simulink model "PVAndBatteryIntegratedPlantForBlackStart"  (R2025b)
settings: Solver=FixedStepAuto  StartTime=0.0  StopTime=tsim  FixedStep=1e-6  RelTol=1e-9  AbsTol=1e-7
InitFcn:
  | %% Black Start Sequence
  | t0 = 0; % Battery IBR initial time
  | t1 = 0.15; % PV IBR initial time
  | t2 = 0.5; % Two IBR sync time
  | t3 = 0.8; % Additional motor load connect
  | t4 = 1.1; % Grid reconnection
  | tsim = 1.5; % Total simulation time
  | 
  | %% initialize
  | Vdc = 400;
  | Vnom = 100;
  | Prated = 10000;
  | Qrated = 0;
  | Srated = sqrt(Prated^2+Qrated^2);
  | wnom = 2*pi*60;
  | fnom = 60;
  | Vminpu = 0.95;
  | 
  | kv = Vnom;
  | ki = 3*Vnom/Srated;
  | 
  | dwmax = 0.5*2*pi;
  | trisemax = 0.1;
  | 
  | C = 1/sqrt(2)/Vminpu^2/dwmax;
  | L = 1/C/wnom^2;
  | tau = C/kv/ki;
  | epsilon = sqrt(L/C);
  | ksy = 3/2/trisemax;
  | 
  | V_voc_1 = 0;
  | V_voc_2 = 0;
  | 
  | % filter
  | Rf = 0.05;
  | Lf = 500e-6;
  | % pwm
  | fsw = 10e3;
  | % simulation
  | Ts = 1e-6;
  | 
  | % load
  | Rl = 3*Vnom^2/Prated;
  | Rl1 = Rl;
  | Rl2 = 2*Rl;
  | Rl3 = 20*Rl;
  | % grid
  | Rg = 0.05;
  | Lg = 50e-6;
  | 
  | % DCDC converter
  | Kp_V = 1;
  | Ki_V = 0.02;
  | Imax = 110;
  | Kp_I = 0.0001;
  | Ki_I = 1;
  | Vcmax = 1;
undefined symbols (not defined in the file): alpha, C_voc, Diode_class, Half_BridgeConverter_class, L_voc, Ll, Mosfet_class, PWMGenerator_DC_DC__class, R_voc, Three_PhaseBreaker_class, Three_PhaseSource_class, Three_PhaseTransformer_2_class, Three_PhaseV_IMeasuremen_class
libraries: nesl_utility x69, ee_lib x49, fl_lib x36, mcbeeMathTransformLib x9, simulink x6, spsParallelRLCBranchLib x3, eePwmGeneratorTwoLevel x2, spsControlledCurrentSourceLib x2, elec_conv_HighZElecRef x2, slpidlib x2, spsSecondOrderFilterLib x1, spsCurrentMeasurementLib x1
(part 1 of 4)
settings Model: SimulationMode=accelerator  Creator=marco  LastModifiedBy=marco
settings DebuggingCC: AlgebraicLoopMsg=none  SaveWithParameterizedLinksMsg=none
settings RTWCC: GPUComputeCapability=3.5

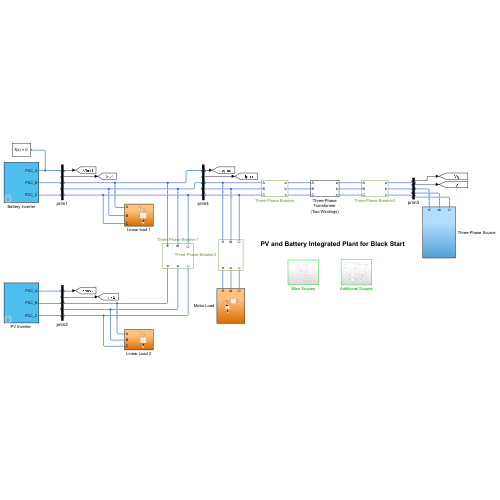
[thumbnail: Simulink's stored preview of the top-level diagram]
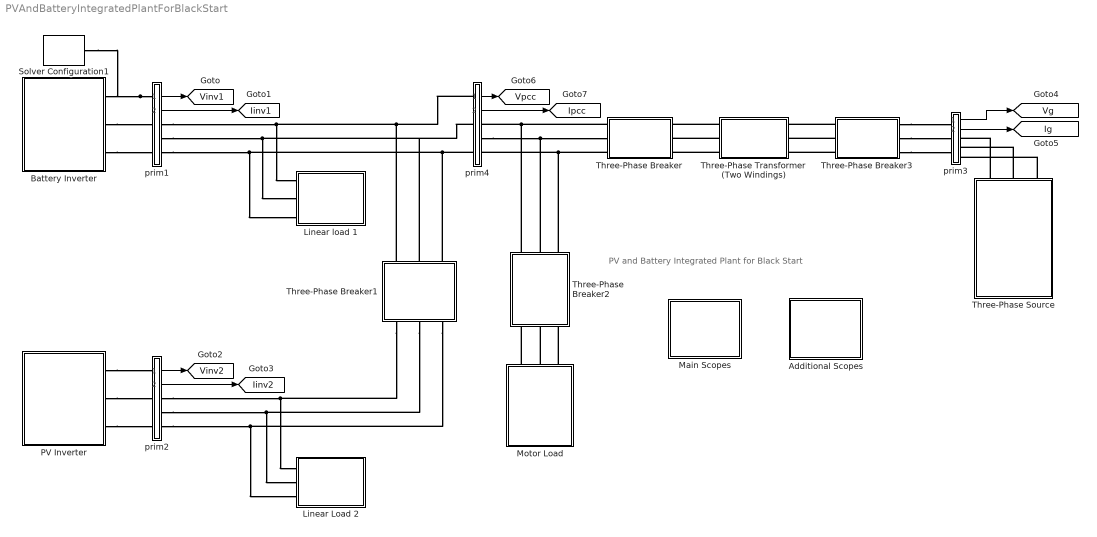
== system PVAndBatteryIntegratedPlantForBlackStart ==
  note: PV and Battery Integrated Plant for Black Start
  Additional Scopes : Subsystem
  Battery Inverter : Subsystem
      mask DialogControl DescTextVar Prompt: This is an IBR with battery source.
  Linear Load 2 : Subsystem
  Linear load 1 : Subsystem
  Main Scopes : Subsystem
  Motor Load : Subsystem
  "PV Inverter " : Subsystem
      mask DialogControl DescTextVar Prompt: This is an IBR with PV source.
  Solver Configuration1 : nesl_utility/Solver Configuration  PhysicalDomain=network_engine_domain  SubClassName=solver  LeftPortType=input  RightPortType=generic  Tones=[]  Harmonics=[]  SimulateNoise=off  Profile=off  UseLocalSampling=off  EnableSwitchedLinearOptims=on  FrequencyDomain=off  UseCCode=off  RelTol=0.001  AbsTol=0.001  MinStep=1e-09  ToWorkspace=off  RevertToSquareIcSolve=off  NumHomotopyIterations=100  PhasorMode=off  PhasorModeNumHarmonics=1  ConsistencySolver=NEWTON_XTOL_AFTER_FTOL  IndexReductionMethod=DerivativeReplacement  DoDC=off  ResidualTolerance=1e-09  ConsistencyTolSource=GLOBAL  ConsistencyAbsTol=0.001  ConsistencyRelTol=0.001  ConsistencyTolFactor=0.001  UseLocalSolver=off  LocalSolverChoice=NE_BACKWARD_EULER_ADVANCER  ResolveIndetEquations=on  FunctionEvalNumThread=1  LocalSolverSampleTime=1e-6  DoFixedCost=on  MaxNonlinIter=3  MaxModeIter=2  ComputeImpulses=off  ImpulseIterations=2  LinearAlgebra=auto  LinearAlgebraNumThread=0  EquationFormulation=NE_TIME_EF  DelaysMemoryBudget=1024  AutomaticFiltering=on  FilteringTimeConstant=0.001  PartitionStorageMethod=AS_NEEDED  PartitionMemoryBudget=1024  PartitionMethod=ROBUST  MultibodyUseLocalSolver=off  MultibodyLocalSolverChoice=ODE1  MultibodyLocalSolverSampleTime=0.001
  Three-Phase Transformer (Two Windings) : Subsystem
      settings: OpenFcn=elec.conv.unmask(gcb);
  Three-Phase Breaker : Subsystem
      settings: OpenFcn=elec.conv.unmask(gcb);
  Three-Phase Breaker1 : Subsystem
      settings: OpenFcn=elec.conv.unmask(gcb);
  Three-Phase Breaker2 : Subsystem
      settings: OpenFcn=elec.conv.unmask(gcb);
  Three-Phase Breaker3 : Subsystem
      settings: OpenFcn=elec.conv.unmask(gcb);
  Three-Phase Source : Subsystem
  prim1 : Subsystem
      settings: OpenFcn=elec.conv.unmask(gcb);
  prim2 : Subsystem
      settings: OpenFcn=elec.conv.unmask(gcb);
  prim3 : Subsystem
      settings: OpenFcn=elec.conv.unmask(gcb);
  prim4 : Subsystem
      settings: OpenFcn=elec.conv.unmask(gcb);
  tag scope: Ig=global, Iinv1=global, Iinv2=global, Ipcc=global, Vg=global, Vinv1=global, Vinv2=global, Vpcc=global
  wires:
  prim1/1(Vabc) -> [Vinv1]
  prim1/2(Iabc) -> [Iinv1]
  prim3/1(Vabc) -> [Vg]
  prim3/2(Iabc) -> [Ig]
  prim2/2(Iabc) -> [Iinv2]
  prim2/1(Vabc) -> [Vinv2]
  prim4/1(Vabc) -> [Vpcc]
  prim4/2(Iabc) -> [Ipcc]
  connections:
  prim1/LConn1 -- Battery Inverter/RConn1 -- Solver Configuration1/RConn1
  Battery Inverter/RConn2 -- prim1/LConn2
  Battery Inverter/RConn3 -- prim1/LConn3
  Three-Phase Breaker1/LConn3 -- prim1/RConn3 -- Linear load 1/LConn3 -- prim4/LConn3
  prim2/RConn1 -- Three-Phase Breaker1/RConn1 -- Linear Load 2/LConn1
  prim2/RConn3 -- Three-Phase Breaker1/RConn3 -- Linear Load 2/LConn3
  "PV Inverter "/RConn3 -- prim2/LConn3
  "PV Inverter "/RConn2 -- prim2/LConn2
  "PV Inverter "/RConn1 -- prim2/LConn1
  Three-Phase Source/RConn1 -- prim3/RConn1
  Three-Phase Source/RConn2 -- prim3/RConn2
  Three-Phase Source/RConn3 -- prim3/RConn3
  Three-Phase Transformer (Two Windings)/LConn2 -- Three-Phase Breaker/RConn2
  Three-Phase Transformer (Two Windings)/LConn1 -- Three-Phase Breaker/RConn1
  Three-Phase Transformer (Two Windings)/LConn3 -- Three-Phase Breaker/RConn3
  Three-Phase Breaker3/RConn2 -- prim3/LConn2
  Three-Phase Breaker3/RConn1 -- prim3/LConn1
  Three-Phase Breaker3/LConn1 -- Three-Phase Transformer (Two Windings)/RConn1
  Three-Phase Breaker3/LConn2 -- Three-Phase Transformer (Two Windings)/RConn2
  Three-Phase Breaker3/LConn3 -- Three-Phase Transformer (Two Windings)/RConn3
  Motor Load/LConn1 -- Three-Phase Breaker2/RConn1
  Motor Load/LConn2 -- Three-Phase Breaker2/RConn2
  Motor Load/LConn3 -- Three-Phase Breaker2/RConn3
  Three-Phase Breaker1/LConn1 -- prim4/LConn1 -- prim1/RConn1 -- Linear load 1/LConn1
  prim2/RConn2 -- Three-Phase Breaker1/RConn2 -- Linear Load 2/LConn2
  Three-Phase Breaker3/RConn3 -- prim3/LConn3
  prim1/RConn2 -- prim4/LConn2 -- Three-Phase Breaker1/LConn2 -- Linear load 1/LConn2
  Three-Phase Breaker2/LConn1 -- Three-Phase Breaker/LConn1 -- prim4/RConn1
  prim4/RConn2 -- Three-Phase Breaker/LConn2 -- Three-Phase Breaker2/LConn2
  Three-Phase Breaker/LConn3 -- prim4/RConn3 -- Three-Phase Breaker2/LConn3

== system PVAndBatteryIntegratedPlantForBlackStart/Additional Scopes ==
  Clarke Transform1 : mcbeeMathTransformLib/Clarke Transform  PowerInvariant=off  UseWithEmbedded=off  PhaseInput=Two inputs
  Clarke Transform2 : mcbeeMathTransformLib/Clarke Transform  PowerInvariant=off  UseWithEmbedded=off  PhaseInput=Two inputs
  Mux : Mux  Inputs=2
  Mux1 : Mux  Inputs=2
  Scope : Scope  NumInputPorts=2
      settings: ActiveDisplayYMinimum=-247.10788  ActiveDisplayYMaximum=247.22597  DataLoggingVariableName=osc_12
  Selector : Selector  InputPortWidth=2  IndexOptions=Index vector (dialog)  Indices=[1]  OutputSizes=1
  Selector1 : Selector  InputPortWidth=3  IndexOptions=Index vector (dialog)  Indices=[1]  OutputSizes=1
  Selector2 : Selector  InputPortWidth=2  IndexOptions=Index vector (dialog)  Indices=[1]  OutputSizes=1
  Selector3 : Selector  InputPortWidth=3  IndexOptions=Index vector (dialog)  Indices=[1]  OutputSizes=1
  wires:
  Clarke Transform1/1 -> Selector1/1
  [Iinv1] -> Clarke Transform1/1
  [V_albe_inv_2] -> Selector/1
  [V_albe_inv_1] -> Selector2/1
  Mux/1 -> Scope/1
  Selector2/1 -> Mux/1
  Selector/1 -> Mux/2
  [Iinv2] -> Clarke Transform2/1
  Clarke Transform2/1 -> Selector3/1
  Selector1/1 -> Mux1/1
  Selector3/1 -> Mux1/2
  Mux1/1 -> Scope/2

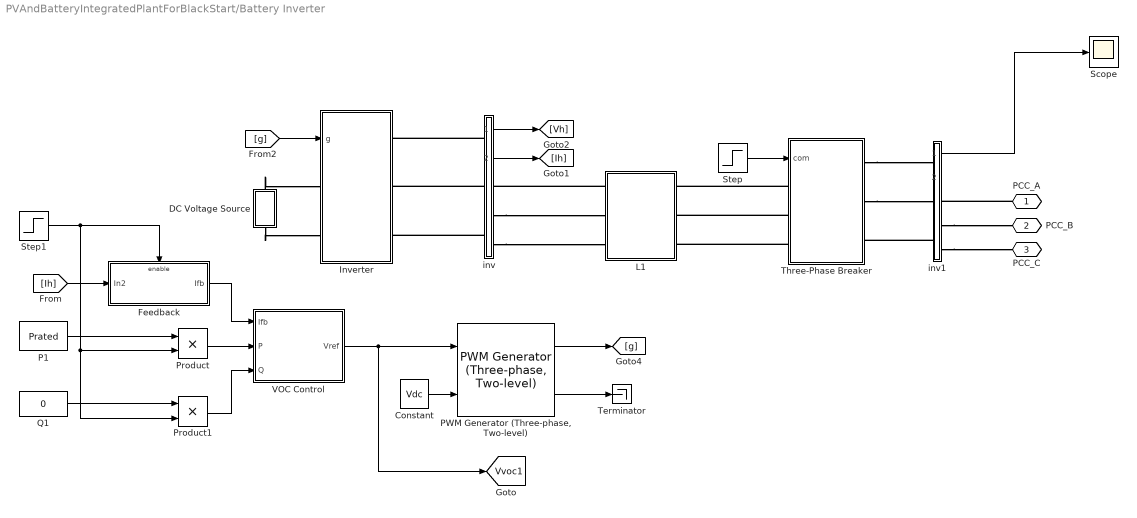
== system PVAndBatteryIntegratedPlantForBlackStart/Battery Inverter ==
  Constant : Constant  Value=Vdc
  DC Voltage Source : Subsystem
      settings: OpenFcn=elec.conv.unmask(gcb);
  Feedback : Subsystem
  Inverter : Subsystem
  L1 : Subsystem
      settings: AttributesFormatString=\n
  P1 : Constant  Value=Prated
  "PWM Generator (Three-phase, Two-level)" : eePwmGeneratorTwoLevel/PWM Generator (Three-phase, Two-level)  PWMMode=Continuous PWM (CPWM)  CPWMMode=SPWM: sinusoidal PWM  DPWMMode=60 DPWM: 60 degree discontinuous PWM  fsw=fsw  Ts=Ts
      settings: LibrarySourceBlock=|
      | ee_sl_lib/Pulse Width
      | Modulation/PWM Generator
      | (Three-phase, Two-level)
  Product : Product
  Product1 : Product
  Q1 : Constant  Value=0
  Scope : Scope
      settings: ActiveDisplayYMinimum=-2.9E-7  ActiveDisplayYMaximum=2E-7  DataLoggingVariableName=ScopeData2
  Step : Step  Time=t0  SampleTime=0
  Step1 : Step  Time=t0  SampleTime=0
  Terminator : Terminator
  Three-Phase Breaker : Subsystem
      settings: OpenFcn=elec.conv.unmask(gcb);
  VOC Control : Subsystem
  inv : Subsystem
      settings: OpenFcn=elec.conv.unmask(gcb);
  inv1 : Subsystem
      settings: OpenFcn=elec.conv.unmask(gcb);
  PCC_A : PMIOPort  Side=Right
  PCC_B : PMIOPort  Port=2  Side=Right
  PCC_C : PMIOPort  Port=3  Side=Right
  tag scope: Vvoc1=global
  wires:
  Q1/1 -> Product1/1
  Product1/1 -> VOC Control/3(Q)
  P1/1 -> Product/1
  Product/1 -> VOC Control/2(P)
  Step1/1 -> Product1/2, Product/2, Feedback/Enable
  Step/1 -> Three-Phase Breaker/1(com)
  Feedback/1(Ifb) -> VOC Control/1(Ifb)
  [g] -> Inverter/1(g)
  Constant/1 -> "PWM Generator (Three-phase, Two-level)"/2
  VOC Control/1(Vref) -> "PWM Generator (Three-phase, Two-level)"/1, [Vvoc1]
  "PWM Generator (Three-phase, Two-level)"/2 -> Terminator/1
  "PWM Generator (Three-phase, Two-level)"/1 -> [g]
  inv/2(Iabc) -> [Ih]
  inv/1(Vabc) -> [Vh]
  [Ih] -> Feedback/1(In2)
  inv1/1(Vabc) -> Scope/1
  connections:
  PCC_A/RConn1 -- inv1/RConn1
  inv1/RConn2 -- PCC_B/RConn1
  inv1/RConn3 -- PCC_C/RConn1
  Three-Phase Breaker/RConn1 -- inv1/LConn1
  Three-Phase Breaker/RConn2 -- inv1/LConn2
  inv1/LConn3 -- Three-Phase Breaker/RConn3
  Three-Phase Breaker/LConn3 -- L1/RConn3
  Three-Phase Breaker/LConn2 -- L1/RConn2
  Three-Phase Breaker/LConn1 -- L1/RConn1
  inv/LConn2 -- Inverter/RConn2
  L1/LConn1 -- inv/RConn1
  DC Voltage Source/RConn1 -- Inverter/LConn1
  inv/LConn3 -- Inverter/RConn3
  DC Voltage Source/LConn1 -- Inverter/LConn2
  inv/RConn3 -- L1/LConn3
  inv/LConn1 -- Inverter/RConn1
  inv/RConn2 -- L1/LConn2

== system PVAndBatteryIntegratedPlantForBlackStart/Linear Load 2 ==
  Ground1 : fl_lib/Electrical/Electrical Elements/Electrical Reference
  Three-Phase Series RLC Branch1 : Subsystem
      settings: AttributesFormatString=\n  OpenFcn=elec.conv.unmask(gcb);
  A : PMIOPort  Side=Left
  B : PMIOPort  Port=2  Side=Left
  C : PMIOPort  Port=3  Side=Left
  connections:
  Three-Phase Series RLC Branch1/RConn3 -- Three-Phase Series RLC Branch1/RConn1 -- Three-Phase Series RLC Branch1/RConn2 -- Ground1/LConn1
  C/RConn1 -- Three-Phase Series RLC Branch1/LConn3
  B/RConn1 -- Three-Phase Series RLC Branch1/LConn2
  A/RConn1 -- Three-Phase Series RLC Branch1/LConn1

== system PVAndBatteryIntegratedPlantForBlackStart/Linear load 1 ==
  Ground : fl_lib/Electrical/Electrical Elements/Electrical Reference
  Three-Phase Series RLC Branch : Subsystem
      settings: AttributesFormatString=\n  OpenFcn=elec.conv.unmask(gcb);
  A : PMIOPort  Side=Left
  B : PMIOPort  Port=2  Side=Left
  C : PMIOPort  Port=3  Side=Left
  connections:
  Three-Phase Series RLC Branch/RConn3 -- Ground/LConn1 -- Three-Phase Series RLC Branch/RConn2 -- Three-Phase Series RLC Branch/RConn1
  A/RConn1 -- Three-Phase Series RLC Branch/LConn1
  C/RConn1 -- Three-Phase Series RLC Branch/LConn3
  B/RConn1 -- Three-Phase Series RLC Branch/LConn2

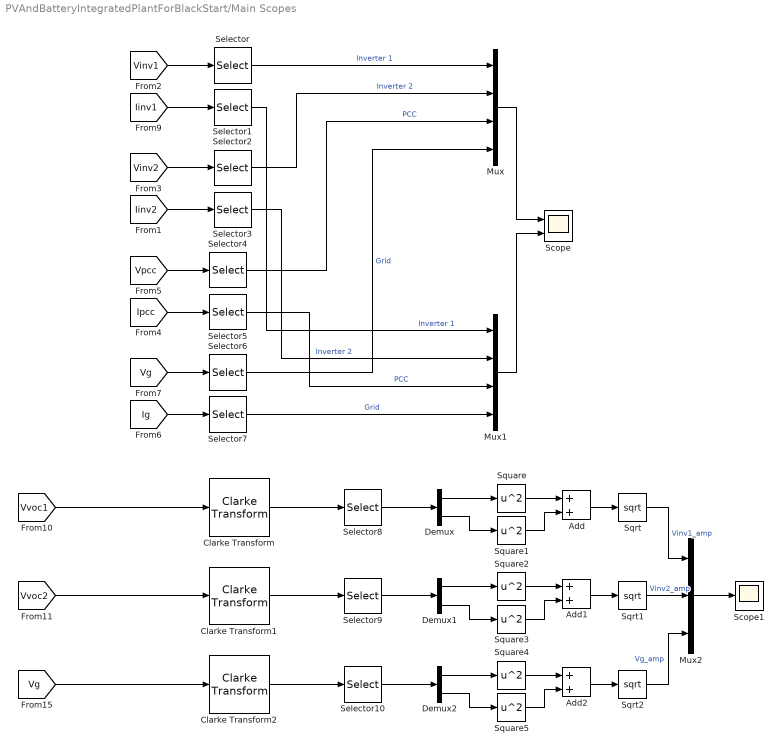
== system PVAndBatteryIntegratedPlantForBlackStart/Main Scopes ==
  Add : Sum
  Add1 : Sum
  Add2 : Sum
  Clarke Transform : mcbeeMathTransformLib/Clarke Transform  PowerInvariant=off  UseWithEmbedded=off  PhaseInput=Two inputs
      settings: LibrarySourceBlock=|
      | ee_sl_lib/Mathematical
      | Transforms/Clarke Transform
  Clarke Transform1 : mcbeeMathTransformLib/Clarke Transform  PowerInvariant=off  UseWithEmbedded=off  PhaseInput=Two inputs
      settings: LibrarySourceBlock=|
      | ee_sl_lib/Mathematical
      | Transforms/Clarke Transform
  Clarke Transform2 : mcbeeMathTransformLib/Clarke Transform  PowerInvariant=off  UseWithEmbedded=off  PhaseInput=Two inputs
      settings: LibrarySourceBlock=|
      | ee_sl_lib/Mathematical
      | Transforms/Clarke Transform
  Demux : Demux  Outputs=2
  Demux1 : Demux  Outputs=2
  Demux2 : Demux  Outputs=2
  Mux : Mux
  Mux1 : Mux
  Mux2 : Mux  Inputs=3
  Scope : Scope  NumInputPorts=2
      settings: ActiveDisplayYMinimum=-60.7192437952104  ActiveDisplayYMaximum=163.88142166690253
  Scope1 : Scope
      settings: ActiveDisplayYMinimum=-24.70319  ActiveDisplayYMaximum=222.32872  DataLoggingVariableName=ScopeData2
  Selector{,1..7} (8 alike) : Selector  InputPortWidth=3  IndexOptions=Index vector (dialog)  Indices=[1]  OutputSizes=1
  Selector10 : Selector  InputPortWidth=3  IndexOptions=Index vector (dialog)  Indices=[1 2]  OutputSizes=1
  Selector8 : Selector  InputPortWidth=3  IndexOptions=Index vector (dialog)  Indices=[1 2]  OutputSizes=1
  Selector9 : Selector  InputPortWidth=3  IndexOptions=Index vector (dialog)  Indices=[1 2]  OutputSizes=1
  Sqrt : Sqrt
  Sqrt1 : Sqrt
  Sqrt2 : Sqrt
  Square{,1..5} (6 alike) : Math  Operator=square
  wires:
  Mux/1 -> Scope/1
  Mux1/1 -> Scope/2
  [Vinv1] -> Selector/1
  [Iinv1] -> Selector1/1
  [Vinv2] -> Selector2/1
  [Iinv2] -> Selector3/1
  [Vpcc] -> Selector4/1
  [Ipcc] -> Selector5/1
  [Vg] -> Selector6/1
  [Ig] -> Selector7/1
  Selector7/1 -> Mux1/4  "Grid"
  Selector6/1 -> Mux/4  "Grid"
  Selector5/1 -> Mux1/3  "PCC"
  Selector3/1 -> Mux1/2  "Inverter 2"
  Selector1/1 -> Mux1/1  "Inverter 1"
  Selector4/1 -> Mux/3  "PCC"
  Selector2/1 -> Mux/2  "Inverter 2"
  Selector/1 -> Mux/1  "Inverter 1"
  [Vvoc1] -> Clarke Transform/1
  [Vg] -> Clarke Transform2/1
  [Vvoc2] -> Clarke Transform1/1
  Clarke Transform/1 -> Selector8/1
  Clarke Transform1/1 -> Selector9/1
  Clarke Transform2/1 -> Selector10/1
  Selector8/1 -> Demux/1
  Demux/1 -> Square/1
  Demux/2 -> Square1/1
  Square/1 -> Add/1
  Square1/1 -> Add/2
  Add/1 -> Sqrt/1
  Square2/1 -> Add1/1
  Add1/1 -> Sqrt1/1
  Square3/1 -> Add1/2
  Demux1/2 -> Square3/1
  Selector9/1 -> Demux1/1
  Demux1/1 -> Square2/1
  Square4/1 -> Add2/1
  Add2/1 -> Sqrt2/1
  Square5/1 -> Add2/2
  Demux2/2 -> Square5/1
  Selector10/1 -> Demux2/1
  Demux2/1 -> Square4/1
  Sqrt1/1 -> Mux2/2  "Vinv2_amp"
  Sqrt/1 -> Mux2/1  "Vinv1_amp"
  Sqrt2/1 -> Mux2/3  "Vg_amp"
  Mux2/1 -> Scope1/1

== system PVAndBatteryIntegratedPlantForBlackStart/Motor Load ==
  Constant : Constant  Value=0
  Ground2 : fl_lib/Electrical/Electrical Elements/Electrical Reference
  Synchronous Machine pu Standard : Subsystem
      settings: OpenFcn=elec.conv.unmask(gcb);
  Terminator : Terminator
  Three-Phase Series RLC Branch3 : Subsystem
      settings: AttributesFormatString=\n  OpenFcn=elec.conv.unmask(gcb);
  A : PMIOPort  Side=Left
  B : PMIOPort  Port=2  Side=Left
  C : PMIOPort  Port=3  Side=Left
  wires:
  Synchronous Machine pu Standard/1(m) -> Terminator/1
  Constant/1 -> Synchronous Machine pu Standard/2(Vf), Synchronous Machine pu Standard/1(Pm)
  connections:
  Three-Phase Series RLC Branch3/RConn3 -- Three-Phase Series RLC Branch3/RConn1 -- Ground2/LConn1 -- Three-Phase Series RLC Branch3/RConn2
  Three-Phase Series RLC Branch3/LConn1 -- A/RConn1 -- Synchronous Machine pu Standard/RConn1
  Synchronous Machine pu Standard/RConn2 -- B/RConn1 -- Three-Phase Series RLC Branch3/LConn2
  Three-Phase Series RLC Branch3/LConn3 -- C/RConn1 -- Synchronous Machine pu Standard/RConn3

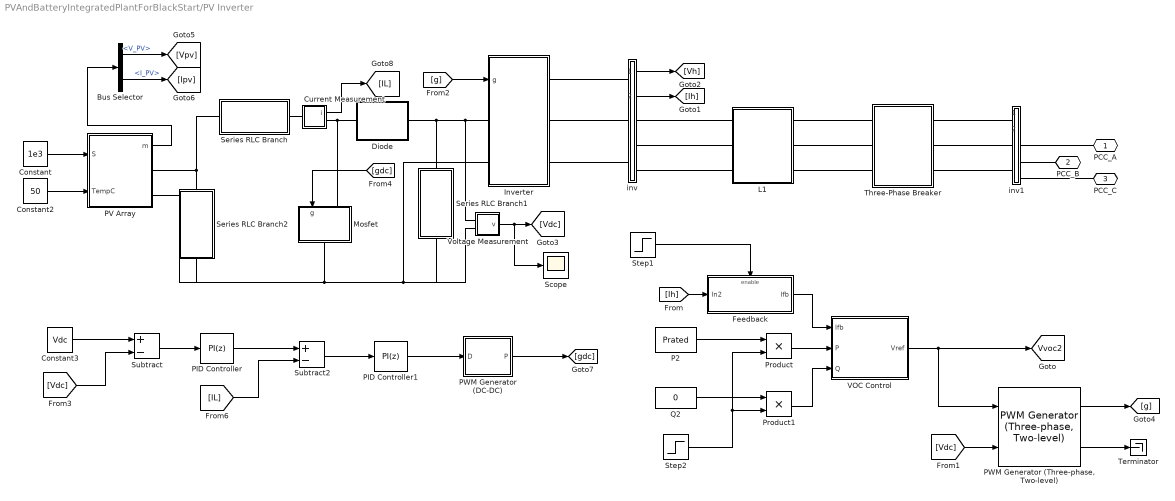
== system PVAndBatteryIntegratedPlantForBlackStart/PV Inverter  ==
  Bus Selector : BusSelector  OutputSignals=V_PV,I_PV
  Constant : Constant  Value=1e3
  Constant2 : Constant  Value=50
  Constant3 : Constant  Value=Vdc
  Current Measurement : Subsystem
      settings: OpenFcn=elec.conv.unmask(gcb);
  Diode : Subsystem
  Feedback : Subsystem
  Inverter : Subsystem
  L1 : Subsystem
      settings: AttributesFormatString=\n  OpenFcn=elec.conv.unmask(gcb);
  Mosfet : Subsystem
      settings: OpenFcn=elec.conv.unmask(gcb);
  P2 : Constant  Value=Prated
  PID Controller : slpidlib/PID Controller  Controller=PI  Form=Parallel  TimeDomain=Discrete-time  UseExternalTs=off  SampleTime=-1  IntegratorMethod=Forward Euler  FilterMethod=Forward Euler  ControllerParametersSource=internal  P=Kp_V  I=Ki_V  UseKiTs=off  D=0  UseExternalDerivativeSource=off  N=100  UseFilter=on  TunerSelectOption=Transfer Function Based (PID Tuner App)  InitialConditionSource=internal  InitialConditionForIntegrator=0  InitialConditionForFilter=0  DifferentiatorICPrevScaledInput=0  ExternalReset=none  TrackingMode=off  Kt=1  LimitOutput=on  SatLimitsSource=internal  UpperSaturationLimit=Imax  LowerSaturationLimit=0  LinearizeAsGain=on  AntiWindupMode=back-calculation  Kb=1  LimitIntegrator=off  UpperIntegratorSaturationLimit=inf  LowerIntegratorSaturationLimit=-inf  POutMin=[]  POutMax=[]  IOutMin=[]  IOutMax=[]  DOutMin=[]  DOutMax=[]  NOutMin=[]  NOutMax=[]  SumOutMin=[]  SumOutMax=[]  SaturationOutMin=[]  SaturationOutMax=[]  PParamMin=[]  PParamMax=[]  IParamMin=[]  IParamMax=[]  DParamMin=[]  DParamMax=[]  NParamMin=[]  NParamMax=[]  KbParamMin=[]  KbParamMax=[]  KtParamMin=[]  KtParamMax=[]  KbOutMin=[]  KbOutMax=[]  KtOutMin=[]  KtOutMax=[]  IntegratorOutMin=[]  IntegratorOutMax=[]  FilterOutMin=[]  FilterOutMax=[]  SumI1OutMin=[]  SumI1OutMax=[]  SumI2OutMin=[]  SumI2OutMax=[]  SumI3OutMin=[]  SumI3OutMax=[]  SumI4OutMin=[]  SumI4OutMax=[]  SumDOutMin=[]  SumDOutMax=[]  DifferentiatorOutMin=[]  DifferentiatorOutMax=[]  FilterDiffOutCoefMin=[]  FilterDiffOutCoefMax=[]  ReciprocalOutMin=[]  ReciprocalOutMax=[]  SumDenOutMin=[]  SumDenOutMax=[]  SumNumOutMin=[]  SumNumOutMax=[]  DivideOutMin=[]  DivideOutMax=[]  UdiffTsProdOutMin=[]  UdiffTsProdOutMax=[]  NTsProdOutMin=[]  NTsProdOutMax=[]  UintegralTsProdOutMin=[]  UintegralTsProdOutMax=[]  UngainTsProdOutMin=[]  UngainTsProdOutMax=[]  ClampingZeroOutDataTypeStr=Inherit: Inherit via back propagation  ClampingZeroOutMin=[]  ClampingZeroOutMax=[]  FilterDenConstantOutDataTypeStr=Inherit: Inherit via back propagation  FilterDenConstantOutMin=[]  FilterDenConstantOutMax=[]  PCopyOutDataTypeStr=Inherit: Inherit via back propagation  PCopyOutMin=[]  PCopyOutMax=[]  NCopyOutDataTypeStr=Inherit: Inherit via back propagation  NCopyOutMin=[]  NCopyOutMax=[]  IntegratorContinuousStateAttributes=''  IntegratorStateMustResolveToSignalObject=off  IntegratorRTWStateStorageClass=Auto  FilterContinuousStateAttributes=''  FilterStateMustResolveToSignalObject=off  FilterRTWStateStorageClass=Auto  ParallelPVariant=InternalParameters  IdealPVariant=Disabled  IVariant=InternalParameters  DVariant=Disabled  IntegratorVariant=Discrete  SatVariant=Enabled  AWVariant=BackCalculation  PCopyVariant=Disabled  TRVariant=Disabled  FdbkBlocksVariant=Forward  IdealPFdbkVariant=Disabled  SatFdbkVariant=Disabled  DerivativeFilterVariant=Disabled  NVariant=Disabled  NCopyVariant=Disabled_SignalSpec  FilterICVariant=Disabled  IntegratorICVariant=InternalICs  ExternalResetVariant=Disabled  TRSumVariant=Passthrough  SumFdbkVariant=Disabled  SumVariant=Sum_PI  TsampFilterVariant=InternalTs  TsampNgainVariant=Passthrough  TsampIntegralVariant=Disabled_SignalSpec  ExternalSaturationOutDataTypeStr=Inherit: Same as second input  DerivativeSourceVariant=Disabled  PreIntVariant=InternalPreInt
  PID Controller1 : slpidlib/PID Controller  Controller=PI  Form=Parallel  TimeDomain=Discrete-time  UseExternalTs=off  SampleTime=-1  IntegratorMethod=Forward Euler  FilterMethod=Forward Euler  ControllerParametersSource=internal  P=Kp_I  I=Ki_I  UseKiTs=off  D=0  UseExternalDerivativeSource=off  N=100  UseFilter=on  TunerSelectOption=Transfer Function Based (PID Tuner App)  InitialConditionSource=internal  InitialConditionForIntegrator=0  InitialConditionForFilter=0  DifferentiatorICPrevScaledInput=0  ExternalReset=none  TrackingMode=off  Kt=1  LimitOutput=on  SatLimitsSource=internal  UpperSaturationLimit=Vcmax  LowerSaturationLimit=0  LinearizeAsGain=on  AntiWindupMode=back-calculation  Kb=1  LimitIntegrator=off  UpperIntegratorSaturationLimit=inf  LowerIntegratorSaturationLimit=-inf  POutMin=[]  POutMax=[]  IOutMin=[]  IOutMax=[]  DOutMin=[]  DOutMax=[]  NOutMin=[]  NOutMax=[]  SumOutMin=[]  SumOutMax=[]  SaturationOutMin=[]  SaturationOutMax=[]  PParamMin=[]  PParamMax=[]  IParamMin=[]  IParamMax=[]  DParamMin=[]  DParamMax=[]  NParamMin=[]  NParamMax=[]  KbParamMin=[]  KbParamMax=[]  KtParamMin=[]  KtParamMax=[]  KbOutMin=[]  KbOutMax=[]  KtOutMin=[]  KtOutMax=[]  IntegratorOutMin=[]  IntegratorOutMax=[]  FilterOutMin=[]  FilterOutMax=[]  SumI1OutMin=[]  SumI1OutMax=[]  SumI2OutMin=[]  SumI2OutMax=[]  SumI3OutMin=[]  SumI3OutMax=[]  SumI4OutMin=[]  SumI4OutMax=[]  SumDOutMin=[]  SumDOutMax=[]  DifferentiatorOutMin=[]  DifferentiatorOutMax=[]  FilterDiffOutCoefMin=[]  FilterDiffOutCoefMax=[]  ReciprocalOutMin=[]  ReciprocalOutMax=[]  SumDenOutMin=[]  SumDenOutMax=[]  SumNumOutMin=[]  SumNumOutMax=[]  DivideOutMin=[]  DivideOutMax=[]  UdiffTsProdOutMin=[]  UdiffTsProdOutMax=[]  NTsProdOutMin=[]  NTsProdOutMax=[]  UintegralTsProdOutMin=[]  UintegralTsProdOutMax=[]  UngainTsProdOutMin=[]  UngainTsProdOutMax=[]  ClampingZeroOutDataTypeStr=Inherit: Inherit via back propagation  ClampingZeroOutMin=[]  ClampingZeroOutMax=[]  FilterDenConstantOutDataTypeStr=Inherit: Inherit via back propagation  FilterDenConstantOutMin=[]  FilterDenConstantOutMax=[]  PCopyOutDataTypeStr=Inherit: Inherit via back propagation  PCopyOutMin=[]  PCopyOutMax=[]  NCopyOutDataTypeStr=Inherit: Inherit via back propagation  NCopyOutMin=[]  NCopyOutMax=[]  IntegratorContinuousStateAttributes=''  IntegratorStateMustResolveToSignalObject=off  IntegratorRTWStateStorageClass=Auto  FilterContinuousStateAttributes=''  FilterStateMustResolveToSignalObject=off  FilterRTWStateStorageClass=Auto  ParallelPVariant=InternalParameters  IdealPVariant=Disabled  IVariant=InternalParameters  DVariant=Disabled  IntegratorVariant=Discrete  SatVariant=Enabled  AWVariant=BackCalculation  PCopyVariant=Disabled  TRVariant=Disabled  FdbkBlocksVariant=Forward  IdealPFdbkVariant=Disabled  SatFdbkVariant=Disabled  DerivativeFilterVariant=Disabled  NVariant=Disabled  NCopyVariant=Disabled_SignalSpec  FilterICVariant=Disabled  IntegratorICVariant=InternalICs  ExternalResetVariant=Disabled  TRSumVariant=Passthrough  SumFdbkVariant=Disabled  SumVariant=Sum_PI  TsampFilterVariant=InternalTs  TsampNgainVariant=Passthrough  TsampIntegralVariant=Disabled_SignalSpec  ExternalSaturationOutDataTypeStr=Inherit: Same as second input  DerivativeSourceVariant=Disabled  PreIntVariant=InternalPreInt
  PV Array : Subsystem
  PWM Generator (DC-DC) : Subsystem
      settings: OpenFcn=elec.conv.unmask(gcb);
  "PWM Generator (Three-phase, Two-level)" : eePwmGeneratorTwoLevel/PWM Generator (Three-phase, Two-level)  PWMMode=Continuous PWM (CPWM)  CPWMMode=SPWM: sinusoidal PWM  DPWMMode=60 DPWM: 60 degree discontinuous PWM  fsw=fsw  Ts=Ts
  Product : Product
  Product1 : Product
  Q2 : Constant  Value=0
  Scope : Scope
      settings: ActiveDisplayYMinimum=-176.21895  ActiveDisplayYMaximum=1586.22409
  Series RLC Branch : Subsystem
      settings: OpenFcn=elec.conv.unmask(gcb);
  Series RLC Branch1 : Subsystem
      settings: OpenFcn=elec.conv.unmask(gcb);
  Series RLC Branch2 : Subsystem
      settings: OpenFcn=elec.conv.unmask(gcb);
  Step1 : Step  Time=t1  SampleTime=0
  Step2 : Step  Time=t1  SampleTime=0
  Subtract : Sum  Inputs=+-
  Subtract2 : Sum  Inputs=+-
  Terminator : Terminator
  Three-Phase Breaker : Subsystem
      settings: OpenFcn=elec.conv.unmask(gcb);
  VOC Control : Subsystem
  Voltage Measurement : Subsystem
      settings: OpenFcn=elec.conv.unmask(gcb);
  inv : Subsystem
      settings: OpenFcn=elec.conv.unmask(gcb);
  inv1 : Subsystem
      settings: OpenFcn=elec.conv.unmask(gcb);
  PCC_A : PMIOPort  Side=Right
  PCC_B : PMIOPort  Port=2  Side=Right
  PCC_C : PMIOPort  Port=3  Side=Right
  tag scope: Vvoc2=global
  wires:
  [Ih] -> Feedback/1(In2)
  inv/1(Vabc) -> [Vh]
  inv/2(Iabc) -> [Ih]
  "PWM Generator (Three-phase, Two-level)"/1 -> [g]
  "PWM Generator (Three-phase, Two-level)"/2 -> Terminator/1
  VOC Control/1(Vref) -> "PWM Generator (Three-phase, Two-level)"/1, [Vvoc2]
  [Vdc] -> "PWM Generator (Three-phase, Two-level)"/2
  [g] -> Inverter/1(g)
  Feedback/1(Ifb) -> VOC Control/1(Ifb)
  Step1/1 -> Feedback/Enable
  Product/1 -> VOC Control/2(P)
  P2/1 -> Product/1
  Product1/1 -> VOC Control/3(Q)
  Q2/1 -> Product1/1
  Step2/1 -> Product/2, Product1/2
  Voltage Measurement/1(v) -> Scope/1, [Vdc]
  Constant/1 -> PV Array/1(S)
  Constant2/1 -> PV Array/2(TempC)
  Bus Selector/1 -> [Vpv]  "<V_PV>"
  Bus Selector/2 -> [Ipv]  "<I_PV>"
  PV Array/1(m) -> Bus Selector/1
  [gdc] -> Mosfet/1(g)
  PWM Generator (DC-DC)/1(P) -> [gdc]
  Constant3/1 -> Subtract/1
  [Vdc] -> Subtract/2
  PID Controller/1 -> Subtract2/1
  [IL] -> Subtract2/2
  Subtract2/1 -> PID Controller1/1
  Subtract/1 -> PID Controller/1
  PID Controller1/1 -> PWM Generator (DC-DC)/1(D)
  Current Measurement/1(i) -> [IL]
  connections:
  inv/RConn2 -- L1/LConn2
  inv/LConn1 -- Inverter/RConn1
  inv/RConn3 -- L1/LConn3
  inv/LConn3 -- Inverter/RConn3
  L1/LConn1 -- inv/RConn1
  inv/LConn2 -- Inverter/RConn2
  Three-Phase Breaker/LConn1 -- L1/RConn1
  Three-Phase Breaker/LConn2 -- L1/RConn2
  Three-Phase Breaker/LConn3 -- L1/RConn3
  inv1/LConn3 -- Three-Phase Breaker/RConn3
  Three-Phase Breaker/RConn2 -- inv1/LConn2
  Three-Phase Breaker/RConn1 -- inv1/LConn1
  inv1/RConn3 -- PCC_C/RConn1
  inv1/RConn2 -- PCC_B/RConn1
  PCC_A/RConn1 -- inv1/RConn1
  Series RLC Branch1/LConn1 -- Voltage Measurement/LConn1 -- Inverter/LConn1 -- Diode/RConn1
  Voltage Measurement/LConn2 -- Series RLC Branch1/RConn1 -- Series RLC Branch2/RConn1 -- PV Array/RConn2 -- Mosfet/RConn1 -- Inverter/LConn2
  Series RLC Branch/LConn1 -- Series RLC Branch2/LConn1 -- PV Array/RConn1
  Mosfet/LConn1 -- Current Measurement/RConn1 -- Diode/LConn1
  Series RLC Branch/RConn1 -- Current Measurement/LConn1

== system PVAndBatteryIntegratedPlantForBlackStart/Three-Phase Transformer (Two Windings) ==
  Two-Winding Transformer (Three-Phase) : ee_lib/Passive/Transformers/Two-Winding Transformer (Three-Phase)  SRated=25000 V*A  FRated=60 Hz  Winding1Connection=3  VRated1=122.5 V  Winding2Connection=3  VRated2=122.5 V  CoreType=2  pu_Rw1=Three_PhaseTransformer_2_class('Yg','Yg','pu',[25000 60],[122.5 0.002 0.08],[122.5 0.002 0.08],500,500,0.5,[0 0;0.0024 1.2;1 1.52],[0.8 -0.8 0.7],'off','off').objParamMappingDerived.NewDerivedParam.pu_Rw1  pu_Rw2=Three_PhaseTransformer_2_class('Yg','Yg','pu',[25000 60],[122.5 0.002 0.08],[122.5 0.002 0.08],500,500,0.5,[0 0;0.0024 1.2;1 1.52],[0.8 -0.8 0.7],'off','off').objParamMappingDerived.NewDerivedParam.pu_Rw2  leakage_reactance_option=ee.enum.transformer_leakage.include  pu_Xl1=Three_PhaseTransformer_2_class('Yg','Yg','pu',[25000 60],[122.5 0.002 0.08],[122.5 0.002 0.08],500,500,0.5,[0 0;0.0024 1.2;1 1.52],[0.8 -0.8 0.7],'off','off').objParamMappingDerived.NewDerivedParam.pu_Xl1  pu_Xl2=Three_PhaseTransformer_2_class('Yg','Yg','pu',[25000 60],[122.5 0.002 0.08],[122.5 0.002 0.08],500,500,0.5,[0 0;0.0024 1.2;1 1.52],[0.8 -0.8 0.7],'off','off').objParamMappingDerived.NewDerivedParam.pu_Xl2  magnetizing_resistance_option=ee.enum.transformer_magnetizingResistance.include  pu_Rm=Three_PhaseTransformer_2_class('Yg','Yg','pu',[25000 60],[122.5 0.002 0.08],[122.5 0.002 0.08],500,500,0.5,[0 0;0.0024 1.2;1 1.52],[0.8 -0.8 0.7],'off','off').objParamMappingDerived.NewDerivedParam.pu_Rm  magnetizing_reactance_option=ee.enum.transformer_magnetizingReactance.include  saturation_option=1  pu_Xm=Three_PhaseTransformer_2_class('Yg','Yg','pu',[25000 60],[122.5 0.002 0.08],[122.5 0.002 0.08],500,500,0.5,[0 0;0.0024 1.2;1 1.52],[0.8 -0.8 0.7],'off','off').objParamMappingDerived.NewDerivedParam.pu_Xm  current_data=Three_PhaseTransformer_2_class('Yg','Yg','pu',[25000 60],[122.5 0.002 0.08],[122.5 0.002 0.08],500,500,0.5,[0 0;0.0024 1.2;1 1.52],[0.8 -0.8 0.7],'off','off').objParamMappingDerived.NewDerivedParam.current_data  magnetic_flux_data=Three_PhaseTransformer_2_class('Yg','Yg','pu',[25000 60],[122.5 0.002 0.08],[122.5 0.002 0.08],500,500,0.5,[0 0;0.0024 1.2;1 1.52],[0.8 -0.8 0.7],'off','off').objParamMappingDerived.NewDerivedParam.magnetic_flux_data  pu_X0=Three_PhaseTransformer_2_class('Yg','Yg','pu',[25000 60],[122.5 0.002 0.08],[122.5 0.002 0.08],500,500,0.5,[0 0;0.0024 1.2;1 1.52],[0.8 -0.8 0.7],'off','off').objParamMappingDerived.NewDerivedParam.pu_X0  i1_specify=off  i1_priority=None  i1=[ 0 0 0 ] A  i1_nominal_specify=off  i1_nominal_value=1  i1_nominal_unit=A  i2_specify=off  i2_priority=None  i2=[ 0 0 0 ] A  i2_nominal_specify=off  i2_nominal_value=1  i2_nominal_unit=A  phi_specify=off  phi_priority=None  phi=Three_PhaseTransformer_2_class('Yg','Yg','pu',[25000 60],[122.5 0.002 0.08],[122.5 0.002 0.08],500,500,0.5,[0 0;0.0024 1.2;1 1.52],[0.8 -0.8 0.7],'off','off').objParamMappingDerived.NewDerivedParam.phi  phi_nominal_specify=off  phi_nominal_value=1  phi_nominal_unit=1  power_dissipated_specify=off  power_dissipated_priority=None  power_dissipated=0 W  power_dissipated_nominal_specify=off  power_dissipated_nominal_value=1  power_dissipated_nominal_unit=W
      settings: InternalSimscapePortConfiguration="{\"Bottom\":[],\"Left\":[{\"id\":\"a1\",\"label\":\"a1\",\"type\":\"foundation.electrical.electrical\"},{\"id\":\"b1\",\"label\":\"b1\",\"type\":\"foundation.electrical.electrical\"},{\"id\":\"c1\",\"label\":\"c1\",\"type\":\"foundation.electrical.electrical\"}],\"Right\":[{\"id\":\"a2\",\"label\":\"a2\",\"type\":\"foundation.electrical.electrical\"},{\"id\":\"b2\",\"label\":\"b2\",\"type\":\"foundation.electrical.electrical\"},{\"id\":\"c2\",\"label\":\"c2\",\"type\":\"foundation.electrical.electrical\"}],\"Top\":[]}"
  A : PMIOPort  Side=Left
  B : PMIOPort  Port=2  Side=Left
  C : PMIOPort  Port=3  Side=Left
  a : PMIOPort  Port=4  Side=Right
  b : PMIOPort  Port=5  Side=Right
  c : PMIOPort  Port=6  Side=Right
  connections:
  A/RConn1 -- Two-Winding Transformer (Three-Phase)/LConn1
  B/RConn1 -- Two-Winding Transformer (Three-Phase)/LConn2
  C/RConn1 -- Two-Winding Transformer (Three-Phase)/LConn3
  Two-Winding Transformer (Three-Phase)/RConn3 -- c/RConn1
  Two-Winding Transformer (Three-Phase)/RConn1 -- a/RConn1
  Two-Winding Transformer (Three-Phase)/RConn2 -- b/RConn1

== system PVAndBatteryIntegratedPlantForBlackStart/Three-Phase Breaker ==
  Circuit Breaker : ee_lib/Switches & Breakers/Circuit Breaker (Three-Phase)  R_closed=0.001 Ohm  G_open=Three_PhaseBreaker_class('open',1000000,Inf,t4,'off').objParamMappingDerived.NewDerivedParam.G_open 1/Ohm  threshold=0.5 V  breaker_behavior=ee.enum.switches.breakerBehavior.zeroCrossingEnable
      settings: InternalSimscapePortConfiguration="{\"Bottom\":[],\"Left\":[{\"id\":\"vT\",\"label\":\"vT\",\"type\":\"input\"},{\"id\":\"a1\",\"label\":\"a1\",\"type\":\"foundation.electrical.electrical\"},{\"id\":\"b1\",\"label\":\"b1\",\"type\":\"foundation.electrical.electrical\"},{\"id\":\"c1\",\"label\":\"c1\",\"type\":\"foundation.electrical.electrical\"}],\"Right\":[{\"id\":\"a2\",\"label\":\"a2\",\"type\":\"foundation.electrical.electrical\"},{\"id\":\"b2\",\"label\":\"b2\",\"type\":\"foundation.electrical.electrical\"},{\"id\":\"c2\",\"label\":\"c2\",\"type\":\"foundation.electrical.electrical\"}],\"Top\":[]}"
  com : Subsystem
  A : PMIOPort  Side=Left
  B : PMIOPort  Port=2  Side=Left
  C : PMIOPort  Port=3  Side=Left
  a : PMIOPort  Port=4  Side=Right
  b : PMIOPort  Port=5  Side=Right
  c : PMIOPort  Port=6  Side=Right
  connections:
  Circuit Breaker/LConn1 -- com/RConn1
  Circuit Breaker/LConn2 -- A/RConn1
  Circuit Breaker/LConn3 -- B/RConn1
  Circuit Breaker/LConn4 -- C/RConn1
  Circuit Breaker/RConn1 -- a/RConn1
  Circuit Breaker/RConn2 -- b/RConn1
  Circuit Breaker/RConn3 -- c/RConn1

== system PVAndBatteryIntegratedPlantForBlackStart/Three-Phase Breaker1 ==
  Circuit Breaker : ee_lib/Switches & Breakers/Circuit Breaker (Three-Phase)  R_closed=0.001 Ohm  G_open=Three_PhaseBreaker_class('open',1000000,Inf,t2,'off').objParamMappingDerived.NewDerivedParam.G_open 1/Ohm  threshold=0.5 V  breaker_behavior=ee.enum.switches.breakerBehavior.zeroCrossingEnable
      settings: InternalSimscapePortConfiguration="{\"Bottom\":[],\"Left\":[{\"id\":\"vT\",\"label\":\"vT\",\"type\":\"input\"},{\"id\":\"a1\",\"label\":\"a1\",\"type\":\"foundation.electrical.electrical\"},{\"id\":\"b1\",\"label\":\"b1\",\"type\":\"foundation.electrical.electrical\"},{\"id\":\"c1\",\"label\":\"c1\",\"type\":\"foundation.electrical.electrical\"}],\"Right\":[{\"id\":\"a2\",\"label\":\"a2\",\"type\":\"foundation.electrical.electrical\"},{\"id\":\"b2\",\"label\":\"b2\",\"type\":\"foundation.electrical.electrical\"},{\"id\":\"c2\",\"label\":\"c2\",\"type\":\"foundation.electrical.electrical\"}],\"Top\":[]}"
  com : Subsystem
  A : PMIOPort  Side=Left
  B : PMIOPort  Port=2  Side=Left
  C : PMIOPort  Port=3  Side=Left
  a : PMIOPort  Port=4  Side=Right
  b : PMIOPort  Port=5  Side=Right
  c : PMIOPort  Port=6  Side=Right
  connections:
  Circuit Breaker/LConn1 -- com/RConn1
  Circuit Breaker/LConn2 -- A/RConn1
  Circuit Breaker/LConn3 -- B/RConn1
  Circuit Breaker/LConn4 -- C/RConn1
  Circuit Breaker/RConn1 -- a/RConn1
  Circuit Breaker/RConn2 -- b/RConn1
  Circuit Breaker/RConn3 -- c/RConn1

== system PVAndBatteryIntegratedPlantForBlackStart/Three-Phase Breaker2 ==
  Circuit Breaker : ee_lib/Switches & Breakers/Circuit Breaker (Three-Phase)  R_closed=0.001 Ohm  G_open=Three_PhaseBreaker_class('open',1000000000,Inf,t3,'off').objParamMappingDerived.NewDerivedParam.G_open 1/Ohm  threshold=0.5 V  breaker_behavior=ee.enum.switches.breakerBehavior.zeroCrossingEnable
      settings: InternalSimscapePortConfiguration="{\"Bottom\":[],\"Left\":[{\"id\":\"vT\",\"label\":\"vT\",\"type\":\"input\"},{\"id\":\"a1\",\"label\":\"a1\",\"type\":\"foundation.electrical.electrical\"},{\"id\":\"b1\",\"label\":\"b1\",\"type\":\"foundation.electrical.electrical\"},{\"id\":\"c1\",\"label\":\"c1\",\"type\":\"foundation.electrical.electrical\"}],\"Right\":[{\"id\":\"a2\",\"label\":\"a2\",\"type\":\"foundation.electrical.electrical\"},{\"id\":\"b2\",\"label\":\"b2\",\"type\":\"foundation.electrical.electrical\"},{\"id\":\"c2\",\"label\":\"c2\",\"type\":\"foundation.electrical.electrical\"}],\"Top\":[]}"
  com : Subsystem
  A : PMIOPort  Side=Left
  B : PMIOPort  Port=2  Side=Left
  C : PMIOPort  Port=3  Side=Left
  a : PMIOPort  Port=4  Side=Right
  b : PMIOPort  Port=5  Side=Right
  c : PMIOPort  Port=6  Side=Right
  connections:
  Circuit Breaker/LConn1 -- com/RConn1
  Circuit Breaker/LConn2 -- A/RConn1
  Circuit Breaker/LConn3 -- B/RConn1
  Circuit Breaker/LConn4 -- C/RConn1
  Circuit Breaker/RConn1 -- a/RConn1
  Circuit Breaker/RConn2 -- b/RConn1
  Circuit Breaker/RConn3 -- c/RConn1

== system PVAndBatteryIntegratedPlantForBlackStart/Three-Phase Breaker3 ==
  Circuit Breaker : ee_lib/Switches & Breakers/Circuit Breaker (Three-Phase)  R_closed=0.001 Ohm  G_open=Three_PhaseBreaker_class('open',1000000,Inf,t4,'off').objParamMappingDerived.NewDerivedParam.G_open 1/Ohm  threshold=0.5 V  breaker_behavior=ee.enum.switches.breakerBehavior.zeroCrossingEnable
      settings: InternalSimscapePortConfiguration="{\"Bottom\":[],\"Left\":[{\"id\":\"vT\",\"label\":\"vT\",\"type\":\"input\"},{\"id\":\"a1\",\"label\":\"a1\",\"type\":\"foundation.electrical.electrical\"},{\"id\":\"b1\",\"label\":\"b1\",\"type\":\"foundation.electrical.electrical\"},{\"id\":\"c1\",\"label\":\"c1\",\"type\":\"foundation.electrical.electrical\"}],\"Right\":[{\"id\":\"a2\",\"label\":\"a2\",\"type\":\"foundation.electrical.electrical\"},{\"id\":\"b2\",\"label\":\"b2\",\"type\":\"foundation.electrical.electrical\"},{\"id\":\"c2\",\"label\":\"c2\",\"type\":\"foundation.electrical.electrical\"}],\"Top\":[]}"
  com : Subsystem
  A : PMIOPort  Side=Left
  B : PMIOPort  Port=2  Side=Left
  C : PMIOPort  Port=3  Side=Left
  a : PMIOPort  Port=4  Side=Right
  b : PMIOPort  Port=5  Side=Right
  c : PMIOPort  Port=6  Side=Right
  connections:
  Circuit Breaker/LConn1 -- com/RConn1
  Circuit Breaker/LConn2 -- A/RConn1
  Circuit Breaker/LConn3 -- B/RConn1
  Circuit Breaker/LConn4 -- C/RConn1
  Circuit Breaker/RConn1 -- a/RConn1
  Circuit Breaker/RConn2 -- b/RConn1
  Circuit Breaker/RConn3 -- c/RConn1

== system PVAndBatteryIntegratedPlantForBlackStart/Three-Phase Source ==
  Electrical Reference : fl_lib/Electrical/Electrical Elements/Electrical Reference
  Voltage Source : ee_lib/Sources/Voltage Source (Three-Phase)  vline_rms=Vnom*sqrt(3) V  shift=0 deg  freq=fnom Hz  impedance_option=0  SShortCircuit=100000000 V*A  XR=7  R=Three_PhaseSource_class(Vnom*sqrt(3),fnom,0,0,100000000,Vnom*sqrt(3),7,'on','off').objParamMappingDerived.NewDerivedParam.R Ohm  L=Three_PhaseSource_class(Vnom*sqrt(3),fnom,0,0,100000000,Vnom*sqrt(3),7,'on','off').objParamMappingDerived.NewDerivedParam.L H  harmonic_option=0  harmonic_orders=[5, 7, 11, 13]  harmonic_ratios=[.1, .1, .1, .1]  G_parasitic=0 1/Ohm  I_specify=off  I_priority=None  I=[ 0 0 0 ] A  I_nominal_specify=off  I_nominal_value=1  I_nominal_unit=A
      settings: InternalSimscapePortConfiguration="{\"Bottom\":[],\"Left\":[{\"id\":\"n\",\"label\":\"n\",\"type\":\"foundation.electrical.electrical\"}],\"Right\":[{\"id\":\"a\",\"label\":\"a\",\"type\":\"foundation.electrical.electrical\"},{\"id\":\"b\",\"label\":\"b\",\"type\":\"foundation.electrical.electrical\"},{\"id\":\"c\",\"label\":\"c\",\"type\":\"foundation.electrical.electrical\"}],\"Top\":[]}"
  A : PMIOPort  Side=Right
  B : PMIOPort  Port=2  Side=Right
  C : PMIOPort  Port=3  Side=Right
  connections:
  Voltage Source/RConn2 -- B/RConn1
  Voltage Source/RConn1 -- A/RConn1
  Voltage Source/RConn3 -- C/RConn1
  Electrical Reference/LConn1 -- Voltage Source/LConn1

== system PVAndBatteryIntegratedPlantForBlackStart/prim1 ==
  Current and Voltage Sensor (Three-Phase) : ee_lib/Sensors & Transducers/Current and Voltage Sensor (Three-Phase)  vMeasurementType=2  outputUnit=2  SRated=100000000 V*A  VRated=500000 V  I_specify=off  I_priority=None  I=[ 0 0 0 ] A  I_nominal_specify=off  I_nominal_value=1  I_nominal_unit=A  V_specify=off  V_priority=None  V=[ 0 0 0 ] V  V_nominal_specify=off  V_nominal_value=1  V_nominal_unit=V
      settings: InternalSimscapePortConfiguration="{\"Bottom\":[],\"Left\":[{\"id\":\"a1\",\"label\":\"a1\",\"type\":\"foundation.electrical.electrical\"},{\"id\":\"b1\",\"label\":\"b1\",\"type\":\"foundation.electrical.electrical\"},{\"id\":\"c1\",\"label\":\"c1\",\"type\":\"foundation.electrical.electrical\"}],\"Right\":[{\"id\":\"V_output\",\"label\":\"V\",\"type\":\"output\"},{\"id\":\"I_output\",\"label\":\"I\",\"type\":\"output\"},{\"id\":\"a2\",\"label\":\"a2\",\"type\":\"foundation.electrical.electrical\"},{\"id\":\"b2\",\"label\":\"b2\",\"type\":\"foundation.electrical.electrical\"},{\"id\":\"c2\",\"label\":\"c2\",\"type\":\"foundation.electrical.electrical\"}],\"Top\":[]}"
  Igain : Gain  Gain=Three_PhaseV_IMeasuremen_class('phase-to-ground','yes','off','off','off',100000000,500000).objParamMappingDerived.NewDerivedParam.IG
  PS-Simulink Converter : nesl_utility/PS-Simulink Converter  PhysicalDomain=network_engine_domain  SubClassName=ps_output  LeftPortType=input  RightPortType=output  PseudoPeriodic=off  Frequencies=[]  VectorFormat=1-D array  Unit=1  AffineConversion=off
  PS-Simulink Converter1 : nesl_utility/PS-Simulink Converter  PhysicalDomain=network_engine_domain  SubClassName=ps_output  LeftPortType=input  RightPortType=output  PseudoPeriodic=off  Frequencies=[]  VectorFormat=1-D array  Unit=1  AffineConversion=off
  Vgain : Gain  Gain=Three_PhaseV_IMeasuremen_class('phase-to-ground','yes','off','off','off',100000000,500000).objParamMappingDerived.NewDerivedParam.VG
  A : PMIOPort  Side=Left
  B : PMIOPort  Port=2  Side=Left
  C : PMIOPort  Port=3  Side=Left
  a : PMIOPort  Port=4  Side=Right
  b : PMIOPort  Port=5  Side=Right
  c : PMIOPort  Port=6  Side=Right
  Vabc : Outport  VectorParamsAs1DForOutWhenUnconnected=off
  Iabc : Outport  Port=2  VectorParamsAs1DForOutWhenUnconnected=off
  wires:
  Igain/1 -> Iabc/1
  Vgain/1 -> Vabc/1
  PS-Simulink Converter1/1 -> Igain/1
  PS-Simulink Converter/1 -> Vgain/1
  connections:
  Current and Voltage Sensor (Three-Phase)/RConn1 -- PS-Simulink Converter/LConn1
  Current and Voltage Sensor (Three-Phase)/RConn2 -- PS-Simulink Converter1/LConn1
  Current and Voltage Sensor (Three-Phase)/RConn5 -- c/RConn1
  Current and Voltage Sensor (Three-Phase)/RConn4 -- b/RConn1
  Current and Voltage Sensor (Three-Phase)/RConn3 -- a/RConn1
  Current and Voltage Sensor (Three-Phase)/LConn3 -- C/RConn1
  Current and Voltage Sensor (Three-Phase)/LConn1 -- A/RConn1
  Current and Voltage Sensor (Three-Phase)/LConn2 -- B/RConn1

== system PVAndBatteryIntegratedPlantForBlackStart/prim2 ==
  Current and Voltage Sensor (Three-Phase) : ee_lib/Sensors & Transducers/Current and Voltage Sensor (Three-Phase)  vMeasurementType=2  outputUnit=2  SRated=100000000 V*A  VRated=500000 V  I_specify=off  I_priority=None  I=[ 0 0 0 ] A  I_nominal_specify=off  I_nominal_value=1  I_nominal_unit=A  V_specify=off  V_priority=None  V=[ 0 0 0 ] V  V_nominal_specify=off  V_nominal_value=1  V_nominal_unit=V
      settings: InternalSimscapePortConfiguration="{\"Bottom\":[],\"Left\":[{\"id\":\"a1\",\"label\":\"a1\",\"type\":\"foundation.electrical.electrical\"},{\"id\":\"b1\",\"label\":\"b1\",\"type\":\"foundation.electrical.electrical\"},{\"id\":\"c1\",\"label\":\"c1\",\"type\":\"foundation.electrical.electrical\"}],\"Right\":[{\"id\":\"V_output\",\"label\":\"V\",\"type\":\"output\"},{\"id\":\"I_output\",\"label\":\"I\",\"type\":\"output\"},{\"id\":\"a2\",\"label\":\"a2\",\"type\":\"foundation.electrical.electrical\"},{\"id\":\"b2\",\"label\":\"b2\",\"type\":\"foundation.electrical.electrical\"},{\"id\":\"c2\",\"label\":\"c2\",\"type\":\"foundation.electrical.electrical\"}],\"Top\":[]}"
  Igain : Gain  Gain=Three_PhaseV_IMeasuremen_class('phase-to-ground','yes','off','off','off',100000000,500000).objParamMappingDerived.NewDerivedParam.IG
  PS-Simulink Converter : nesl_utility/PS-Simulink Converter  PhysicalDomain=network_engine_domain  SubClassName=ps_output  LeftPortType=input  RightPortType=output  PseudoPeriodic=off  Frequencies=[]  VectorFormat=1-D array  Unit=1  AffineConversion=off
  PS-Simulink Converter1 : nesl_utility/PS-Simulink Converter  PhysicalDomain=network_engine_domain  SubClassName=ps_output  LeftPortType=input  RightPortType=output  PseudoPeriodic=off  Frequencies=[]  VectorFormat=1-D array  Unit=1  AffineConversion=off
  Vgain : Gain  Gain=Three_PhaseV_IMeasuremen_class('phase-to-ground','yes','off','off','off',100000000,500000).objParamMappingDerived.NewDerivedParam.VG
  A : PMIOPort  Side=Left
  B : PMIOPort  Port=2  Side=Left
  C : PMIOPort  Port=3  Side=Left
  a : PMIOPort  Port=4  Side=Right
  b : PMIOPort  Port=5  Side=Right
  c : PMIOPort  Port=6  Side=Right
  Vabc : Outport  VectorParamsAs1DForOutWhenUnconnected=off
  Iabc : Outport  Port=2  VectorParamsAs1DForOutWhenUnconnected=off
  wires:
  Igain/1 -> Iabc/1
  Vgain/1 -> Vabc/1
  PS-Simulink Converter1/1 -> Igain/1
  PS-Simulink Converter/1 -> Vgain/1
  connections:
  Current and Voltage Sensor (Three-Phase)/RConn1 -- PS-Simulink Converter/LConn1
  Current and Voltage Sensor (Three-Phase)/RConn2 -- PS-Simulink Converter1/LConn1
  Current and Voltage Sensor (Three-Phase)/RConn5 -- c/RConn1
  Current and Voltage Sensor (Three-Phase)/RConn4 -- b/RConn1
  Current and Voltage Sensor (Three-Phase)/RConn3 -- a/RConn1
  Current and Voltage Sensor (Three-Phase)/LConn3 -- C/RConn1
  Current and Voltage Sensor (Three-Phase)/LConn1 -- A/RConn1
  Current and Voltage Sensor (Three-Phase)/LConn2 -- B/RConn1

== system PVAndBatteryIntegratedPlantForBlackStart/prim3 ==
  Current and Voltage Sensor (Three-Phase) : ee_lib/Sensors & Transducers/Current and Voltage Sensor (Three-Phase)  vMeasurementType=2  outputUnit=2  SRated=100000000 V*A  VRated=500000 V  I_specify=off  I_priority=None  I=[ 0 0 0 ] A  I_nominal_specify=off  I_nominal_value=1  I_nominal_unit=A  V_specify=off  V_priority=None  V=[ 0 0 0 ] V  V_nominal_specify=off  V_nominal_value=1  V_nominal_unit=V
      settings: InternalSimscapePortConfiguration="{\"Bottom\":[],\"Left\":[{\"id\":\"a1\",\"label\":\"a1\",\"type\":\"foundation.electrical.electrical\"},{\"id\":\"b1\",\"label\":\"b1\",\"type\":\"foundation.electrical.electrical\"},{\"id\":\"c1\",\"label\":\"c1\",\"type\":\"foundation.electrical.electrical\"}],\"Right\":[{\"id\":\"V_output\",\"label\":\"V\",\"type\":\"output\"},{\"id\":\"I_output\",\"label\":\"I\",\"type\":\"output\"},{\"id\":\"a2\",\"label\":\"a2\",\"type\":\"foundation.electrical.electrical\"},{\"id\":\"b2\",\"label\":\"b2\",\"type\":\"foundation.electrical.electrical\"},{\"id\":\"c2\",\"label\":\"c2\",\"type\":\"foundation.electrical.electrical\"}],\"Top\":[]}"
  Igain : Gain  Gain=Three_PhaseV_IMeasuremen_class('phase-to-ground','yes','off','off','off',100000000,500000).objParamMappingDerived.NewDerivedParam.IG
  PS-Simulink Converter : nesl_utility/PS-Simulink Converter  PhysicalDomain=network_engine_domain  SubClassName=ps_output  LeftPortType=input  RightPortType=output  PseudoPeriodic=off  Frequencies=[]  VectorFormat=1-D array  Unit=1  AffineConversion=off
  PS-Simulink Converter1 : nesl_utility/PS-Simulink Converter  PhysicalDomain=network_engine_domain  SubClassName=ps_output  LeftPortType=input  RightPortType=output  PseudoPeriodic=off  Frequencies=[]  VectorFormat=1-D array  Unit=1  AffineConversion=off
  Vgain : Gain  Gain=Three_PhaseV_IMeasuremen_class('phase-to-ground','yes','off','off','off',100000000,500000).objParamMappingDerived.NewDerivedParam.VG
  A : PMIOPort  Side=Left
  B : PMIOPort  Port=2  Side=Left
  C : PMIOPort  Port=3  Side=Left
  a : PMIOPort  Port=4  Side=Right
  b : PMIOPort  Port=5  Side=Right
  c : PMIOPort  Port=6  Side=Right
  Vabc : Outport  VectorParamsAs1DForOutWhenUnconnected=off
  Iabc : Outport  Port=2  VectorParamsAs1DForOutWhenUnconnected=off
  wires:
  Igain/1 -> Iabc/1
  Vgain/1 -> Vabc/1
  PS-Simulink Converter1/1 -> Igain/1
  PS-Simulink Converter/1 -> Vgain/1
  connections:
  Current and Voltage Sensor (Three-Phase)/RConn1 -- PS-Simulink Converter/LConn1
  Current and Voltage Sensor (Three-Phase)/RConn2 -- PS-Simulink Converter1/LConn1
  Current and Voltage Sensor (Three-Phase)/RConn5 -- c/RConn1
  Current and Voltage Sensor (Three-Phase)/RConn4 -- b/RConn1
  Current and Voltage Sensor (Three-Phase)/RConn3 -- a/RConn1
  Current and Voltage Sensor (Three-Phase)/LConn3 -- C/RConn1
  Current and Voltage Sensor (Three-Phase)/LConn1 -- A/RConn1
  Current and Voltage Sensor (Three-Phase)/LConn2 -- B/RConn1
